simulink model "Simulator2"  (R2017b)
settings: Solver=VariableStepAuto  StartTime=0.0  StopTime=10.0  RelTol=1e-3
libraries: simulink_extras x2
settings Model: Creator=gu.marugan-rubio  LastModifiedBy=gu.marugan-rubio

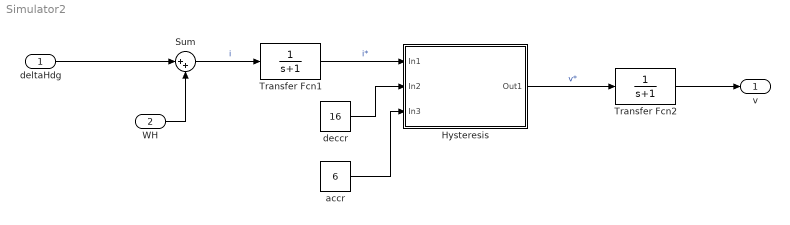
== system Simulator2 ==
  deltaHdg : Inport
  WH : Inport  Port=2
  "Hysteresis " : Subsystem
  Sum : Sum  Inputs=|++
  Transfer Fcn1 : TransferFcn  Denominator=[1 1]
  Transfer Fcn2 : TransferFcn  Denominator=[1 1]
  accr : Constant  Value=6
  deccr : Constant  Value=16
  v : Outport
  wires:
  deccr/1 -> "Hysteresis "/2(In2)
  accr/1 -> "Hysteresis "/3(In3)
  Transfer Fcn1/1 -> "Hysteresis "/1(In1)  "i*"
  "Hysteresis "/1(Out1) -> Transfer Fcn2/1  "v*"
  Transfer Fcn2/1 -> v/1
  deltaHdg/1 -> Sum/1
  Sum/1 -> Transfer Fcn1/1  "i"
  WH/1 -> Sum/2

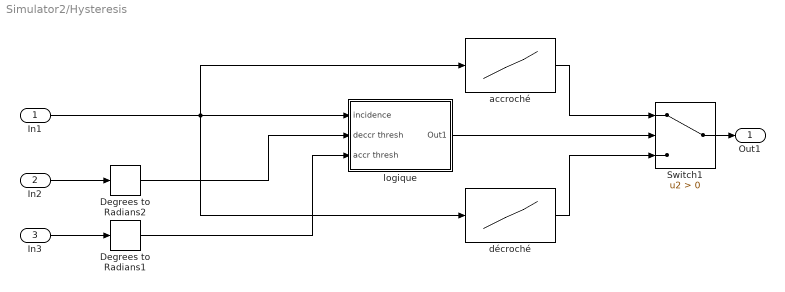
== system Simulator2/Hysteresis  ==
  In1 : Inport
  In2 : Inport  Port=2
  In3 : Inport  Port=3
  Degrees to Radians1 : simulink_extras/Transformations/Degrees to Radians
  Degrees to Radians2 : simulink_extras/Transformations/Degrees to Radians
  Switch1 : Switch  Criteria=u2 > Threshold
  accroché : Lookup  InputValues=[0;2;4;6;8;10;12;14]*pi/180  Table=[0;0.112533129751682;0.223609894514084;0.332737416028976;0.453826665878296;0.563470125198364;0.661327242851257;0.728185296058655]  SaturateOnIntegerOverflow=on
  décroché : Lookup  InputValues=|  Table=|  SaturateOnIntegerOverflow=on
      InputValues=|
      | [0
      |      2
      |      4
      |      6
      |      8
      |     10
      |     12
      |     14
      |     16
      |     18
      |     20
      |     22
      |     24
      |     26
      |     28
      |     30]*pi/180
      Table=|
      | [0
      |     0.1075
      |     0.2196
      |     0.3391
      |     0.3905
      |     0.3900
      |     0.4267
      |     0.4251
      |     0.4248
      |     0.4398
      |     0.4567
      |     0.4783
      |     0.4959
      |     0.5121
      |     0.5003
      |     0.5181]
  logique : Subsystem
  Out1 : Outport
  wires:
  Switch1/1 -> Out1/1
  In3/1 -> Degrees to Radians1/1
  Degrees to Radians2/1 -> logique/2(deccr thresh)
  In1/1 -> décroché/1, accroché/1, logique/1("incidence ")
  accroché/1 -> Switch1/1
  Degrees to Radians1/1 -> logique/3(accr thresh)
  In2/1 -> Degrees to Radians2/1
  décroché/1 -> Switch1/3
  logique/1(Out1) -> Switch1/2

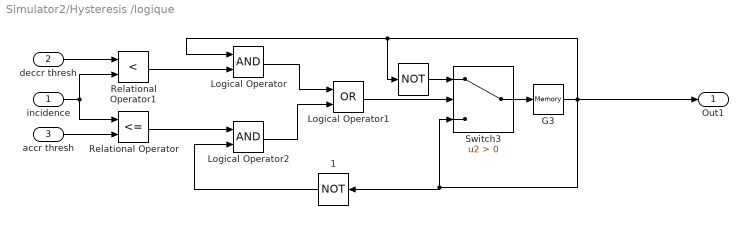
== system Simulator2/Hysteresis /logique ==
  "incidence " : Inport
  deccr thresh : Inport  Port=2
  accr thresh : Inport  Port=3
  " " : Logic  Operator=NOT  AllPortsSameDT=off  OutDataTypeStr=boolean
  " 1" : Logic  Operator=NOT  AllPortsSameDT=off  OutDataTypeStr=boolean
  G3 : Memory  InitialCondition=1
  Logical Operator : Logic  AllPortsSameDT=off  OutDataTypeStr=boolean
  Logical Operator1 : Logic  Operator=OR  AllPortsSameDT=off  OutDataTypeStr=boolean
  Logical Operator2 : Logic  AllPortsSameDT=off  OutDataTypeStr=boolean
  Relational Operator : RelationalOperator  Operator=<=  OutDataTypeStr=boolean  RndMeth=Simplest
  Relational Operator1 : RelationalOperator  Operator=<  OutDataTypeStr=boolean  RndMeth=Simplest
  Switch3 : Switch  Criteria=u2 > Threshold
  Out1 : Outport
  wires:
  Switch3/1 -> G3/1
  accr thresh/1 -> Relational Operator/2
  "incidence "/1 -> Relational Operator/1, Relational Operator1/2
  deccr thresh/1 -> Relational Operator1/1
  G3/1 -> Switch3/3, " 1"/1, Out1/1, Logical Operator/1, " "/1
  " "/1 -> Switch3/1
  Relational Operator1/1 -> Logical Operator/2
  Logical Operator1/1 -> Switch3/2
  Logical Operator/1 -> Logical Operator1/1
  Logical Operator2/1 -> Logical Operator1/2
  Relational Operator/1 -> Logical Operator2/1
  " 1"/1 -> Logical Operator2/2
